simulink library "pkg"  (Simulink 8.1)
settings: Solver=ode45  StartTime=0.0  StopTime=10.0  RelTol=1e-3
undefined symbols (not defined in the file or in its folder): C_TICK_TIME_S, ENUM_GEARPOSN_PN, ENUM_GEARPOSN_R, ENUM_PARKBRAKEBINDSTA_TIGHTENED, FALSE, KIFO_ParkingSituationTimer_ms, KIFO_SteeringAngleParking_deg, TRUE
libraries: hcu_lib x1
settings Model: Creator=xsellart  LastModifiedBy=AT015555

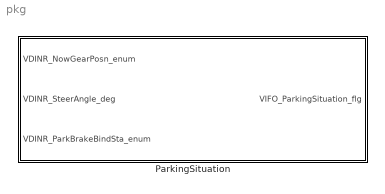
== system pkg ==
  ParkingSituation : Subsystem

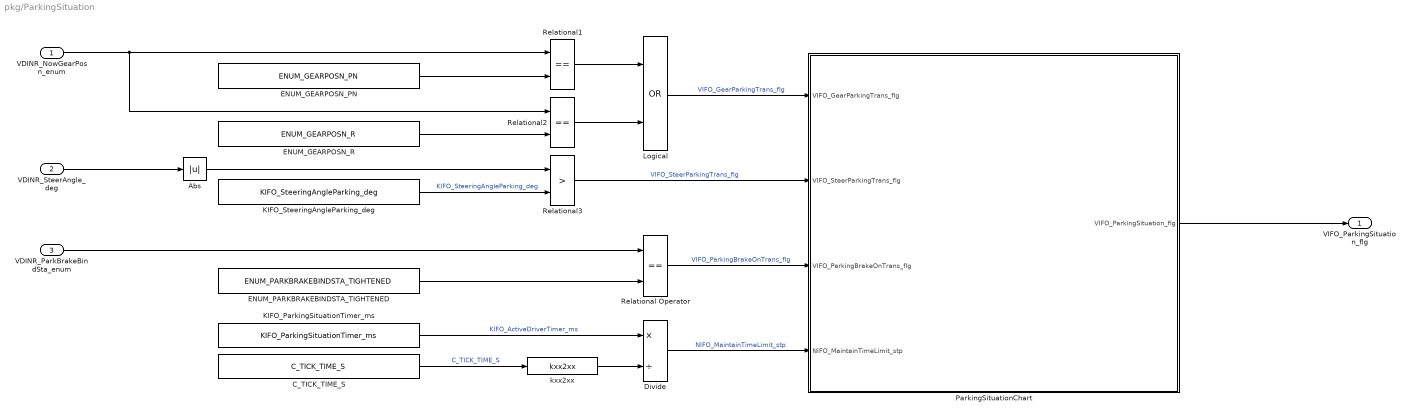
== system pkg/ParkingSituation ==
  VDINR_NowGearPosn_enum : Inport
  VDINR_SteerAngle_deg : Inport  Port=2
  VDINR_ParkBrakeBindSta_enum : Inport  Port=3
  Abs : Abs
  C_TICK_TIME_S : Constant  Value=C_TICK_TIME_S  OutDataTypeStr=single
  Divide : Product  Inputs=*/
  ENUM_GEARPOSN_PN : Constant  Value=ENUM_GEARPOSN_PN  OutDataTypeStr=uint8
  ENUM_GEARPOSN_R : Constant  Value=ENUM_GEARPOSN_R  OutDataTypeStr=uint8
  ENUM_PARKBRAKEBINDSTA_TIGHTENED : Constant  Value=ENUM_PARKBRAKEBINDSTA_TIGHTENED  OutDataTypeStr=uint8
  KIFO_ParkingSituationTimer_ms : Constant  Value=KIFO_ParkingSituationTimer_ms  OutDataTypeStr=single
  KIFO_SteeringAngleParking_deg : Constant  Value=KIFO_SteeringAngleParking_deg  OutDataTypeStr=single
  Logical : Logic  Operator=OR  AllPortsSameDT=off  OutDataTypeStr=boolean
  ParkingSituationChart : Stateflow chart  TreatAsAtomicUnit=on
  Relational Operator : RelationalOperator  Operator===  OutDataTypeStr=boolean
  Relational1 : RelationalOperator  Operator===  OutDataTypeStr=boolean
  Relational2 : RelationalOperator  Operator===  OutDataTypeStr=boolean
  Relational3 : RelationalOperator  Operator=>  OutDataTypeStr=boolean
  kxx2xx : hcu_lib/kxx2xx
  VIFO_ParkingSituation_flg : Outport
  wires:
  ENUM_PARKBRAKEBINDSTA_TIGHTENED/1 -> Relational Operator/2
  Relational Operator/1 -> ParkingSituationChart/3(VIFO_ParkingBrakeOnTrans_flg)  "VIFO_ParkingBrakeOnTrans_flg"
  VDINR_ParkBrakeBindSta_enum/1 -> Relational Operator/1
  kxx2xx/1 -> Divide/2
  C_TICK_TIME_S/1 -> kxx2xx/1  "C_TICK_TIME_S"
  Abs/1 -> Relational3/1
  Divide/1 -> ParkingSituationChart/4(NIFO_MaintainTimeLimit_stp)  "NIFO_MaintainTimeLimit_stp"
  KIFO_ParkingSituationTimer_ms/1 -> Divide/1  "KIFO_ActiveDriverTimer_ms"
  ParkingSituationChart/1(VIFO_ParkingSituation_flg) -> VIFO_ParkingSituation_flg/1
  Relational3/1 -> ParkingSituationChart/2(VIFO_SteerParkingTrans_flg)  "VIFO_SteerParkingTrans_flg"
  Logical/1 -> ParkingSituationChart/1(VIFO_GearParkingTrans_flg)  "VIFO_GearParkingTrans_flg"
  KIFO_SteeringAngleParking_deg/1 -> Relational3/2  "KIFO_SteeringAngleParking_deg"
  VDINR_SteerAngle_deg/1 -> Abs/1
  Relational2/1 -> Logical/2
  Relational1/1 -> Logical/1
  ENUM_GEARPOSN_R/1 -> Relational2/2
  ENUM_GEARPOSN_PN/1 -> Relational1/2
  VDINR_NowGearPosn_enum/1 -> Relational1/1, Relational2/1

== stateflow chart ParkingSituation/ParkingSituationChart ==
  state DRIVING
    en:
    VIFO_ParkingSituation_flg = FALSE;
  state PARKING
    en:
    VIFO_ParkingSituation_flg = TRUE;
  state MAINTAIN
    en:
    NIFO_MaintainTimeLocal_stp = 0;
    du:
    NIFO_MaintainTimeLocal_stp = NIFO_MaintainTimeLocal_stp +1;
  (default) -> DRIVING
  (junction 14) -> DRIVING : [NIFO_MaintainTimeLocal_stp > NIFO_MaintainTimeLimit_stp]
  MAINTAIN -> (junction 14) [order 2]
  DRIVING -> (junction 15)
  PARKING -> MAINTAIN : [VIFO_GearParkingTrans_flg==FALSE ...
      | && VIFO_SteerParkingTrans_flg==FALSE ...
      | && VIFO_ParkingBrakeOnTrans_flg==FALSE]
  (junction 15) -> PARKING : [VIFO_GearParkingTrans_flg==TRUE ...
      | || VIFO_SteerParkingTrans_flg==TRUE ...
      | || VIFO_ParkingBrakeOnTrans_flg==TRUE]
  MAINTAIN -> PARKING [order 1] : [VIFO_GearParkingTrans_flg==TRUE ...
      | || VIFO_SteerParkingTrans_flg==TRUE ...
      | || VIFO_ParkingBrakeOnTrans_flg==TRUE]
  data: VIFO_ParkingSituation_flg output boolean; VIFO_GearParkingTrans_flg input boolean; VIFO_SteerParkingTrans_flg input boolean; VIFO_ParkingBrakeOnTrans_flg input boolean; TRUE parameter boolean; FALSE parameter double; NIFO_MaintainTimeLocal_stp local single; NIFO_MaintainTimeLimit_stp input single
